simulink model "Loop_detailed_model_comp_cc_vccc_v14_JAWOLL_2"  (R2013a)
settings: Solver=ode15s  SolverMode=SingleTasking  StartTime=0.0  StopTime=8e-3  FixedStep=FS  MaxStep=1e-4  RelTol=1e-3
PreLoadFcn:
  | %lowerVoltageLimit=str2num(get_param(gcs,'lowerVoltageLimit'));
  | %upperVoltageLimit=str2num(get_param(gcs,'upperVoltageLimit'));
InitFcn:
  | %%%%%%  set scope time range
  | T_STOP=str2num(get_param(gcs,'StopTime'));
  | if numel(T_STOP) > 1
  |    T_STOP=T_STOP(2);
  | else
  |    T_STOP=T_STOP(1);
  | end
  | T_STOP=num2str(T_STOP);
  | 
  | %%%%%%  set scope time range in system @init_callback_fct
  | T_STOP=num2str(str2num(get_param(gcs,'StopTime')));
  | 
  | childs = allchild(0);
  | sol=strfind(upper(get(allchild(0),'Tag')),'VIEWER_PARAMETERS');
  | 
  | if iscell(sol)
  |    ind=find(~cellfun(@isempty, strfind(upper(get(allchild(0),'Tag')),'VIEWER_PARAMETERS')));
  | else
  |    ind=sol;
  | end
  | %ind=find(~cellfun(@isempty, {strfind(upper(get(allchild(0),'Tag')),'VIEWER_PARAMETERS'),[]}))
  | if ~isempty(ind)
  |    for k=1:length(childs(ind))
  |       set_param(getfield(get(childs(ind(k)),'UserData'),'block'),'TimeRange', T_STOP);
  | %      get_param(getfield(get(childs(ind(k)),'UserData'),'block'),'TimeRange');
  | %    set_param(getfield(get(childs(ind),'UserData'),'block'),'TimeRange',T_STOP);
  | %    get_param(getfield(get(childs(ind),'UserData'),'block'),'TimeRange');
  |    end
  | else
  |     warning(sprintf('VIEWER_PARAMETERS object not found\nOpen the config dialog by hand for the first sim start'))
  | end
StartFcn:
  | lowerVoltageLimit=str2num(get_param(gcs,'lowerVoltageLimit'));
  | upperVoltageLimit=str2num(get_param(gcs,'upperVoltageLimit'));
model workspace (MATLAB code in the model file):
  | lowerVoltageLimit=str2num(get_param(gcs,'lowerVoltageLimit'));
  | upperVoltageLimit=str2num(get_param(gcs,'upperVoltageLimit'));
values from neighbouring files (symbols this model uses):
  FS = 5e-6    (= 5e-06)    [GalvoModel_v4_sys.m]    (also in GalvoModel_v6_sys.m = 5e-05; Galvo_process_analyze.m = 0.0001)
  Lc = 170e-6    (= 0.00017)    [GalvoModel_v6_sys.m]    (also in Galvo_process_analyze.m)
undefined symbols (not defined in the file or in its folder): ccG0
libraries: simulink x2
settings Model: upperVoltageLimit=30  lowerVoltageLimit=-30  BufferReuse=off  Creator=mainster  LastModifiedBy=mainster
settings SolverCC: AutoInsertRateTranBlk=on
settings OptimizationCC: InlineParams=on  BufferReuse=off
settings DebuggingCC: InitInArrayFormatMsg=none
settings HardwareCC: ProdLargestAtomicInteger=Long  ProdLargestAtomicFloat=Double  ProdEndianess=LittleEndian  ProdHWDeviceType=ARM Compatible->ARM Cortex

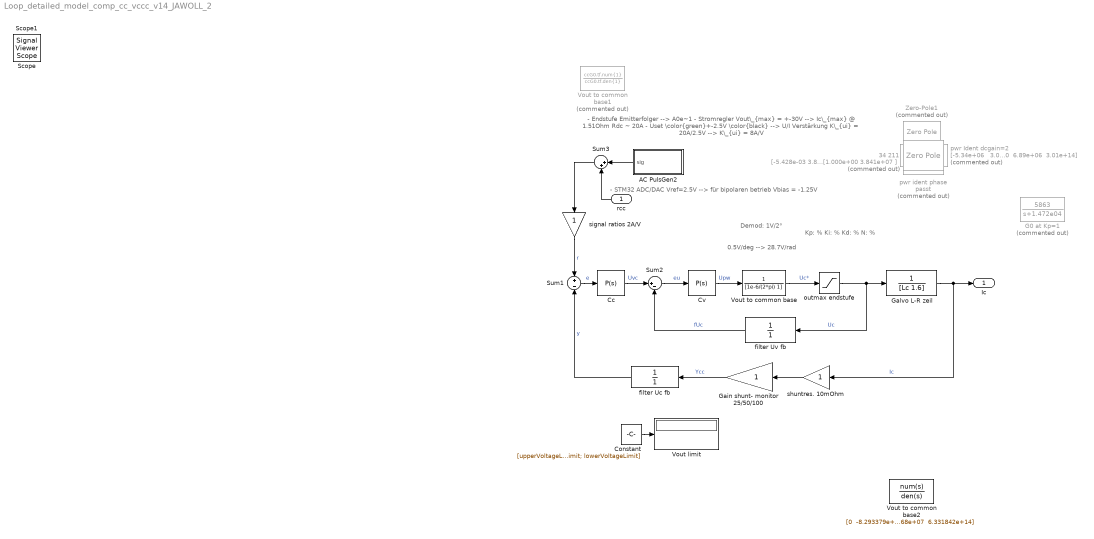
== system Loop_detailed_model_comp_cc_vccc_v14_JAWOLL_2 ==
  note: - Endstufe Emitterfolger --> A0e~1
      | - Stromregler Vout\_{max} = +-30V
      |       --> Ic\_{max} @ 1.51Ohm Rdc ~ 20A
      | - Uset \color{green}+-2.5V \color{black}
      |       --> U/I Verstärkung K\_{ui} = 20A/2.5V
      |       --> K\_{ui} = 8A/V
  note: - STM32 ADC/DAC Vref=2.5V
      | --> für bipolaren betrieb Vbias = -1.25V
  note: Kp: % Ki: % Kd: % N: %
  note: 0.5V/deg --> 28.7V/rad
  note: Demod:
      | 1V/2°
  rcc : Inport
  34 211 : TransferFcn  Commented=on  Numerator=[-5.428e-03 3.828e+07 ]/[-5.428e-03 3.828e+07 ]  Denominator=[1.000e+00 3.841e+07 ]/[1.000e+00 3.841e+07 ]
  AC PulsGen2 : Subsystem  mask{sigp=1, sigpp=0, offs=0}
      mask prompts: sigp "Insert signal peak"; sigpp "or signal peak-to-peak"; offs "Insert DC offset"
      mask TypeOptions sigp: PulsGen/Amplitude
      mask Callback sigp:
      | %sigp=get_param([gcb '/PulsGen'],'Amplitude')
      | %SigVal=2*sigp
      mask TypeOptions offs: offset/Value
      mask Display:
      | %str=sprintf('%s',get(gcbh,'ModelName'));
      | port_label('output', 1, '','texmode','off')
      | %text(.05,.98,['{\fontsize{12}\it\bf' strrep(str,'_',' ') '}'],'horizontalAlignment','left','verticalAlignment','top','texmode','on')
      | %text(.5,0.95,['{\fontsize{8}A_{peak}=}'],'horizontalAlignment','center','verticalAlignment','top','texmode','on')
      | disp(sprintf('Up=%.3g\nDC=%.3g',sigp, offs))
      | %disp(['Upp=' sigpp])%, offs))
      | %sprintf('sigpp==%s',sigpp)
      | %text(.15,.05,['{\fontsize{10}\itmechanics}'],'horizontalAlignment','left','verticalAlignment','bottom','texmode','on')
  Cc : simulink/Continuous/PID Controller  Controller=P  TimeDomain=Continuous-time  SampleTime=1  IntegratorMethod=Forward Euler  FilterMethod=Forward Euler  Form=Parallel  P=10  I=1  D=0  N=100  InitialConditionSource=internal  InitialConditionForIntegrator=0  InitialConditionForFilter=0  ExternalReset=none  LimitOutput=on  UpperSaturationLimit=30  LowerSaturationLimit=-30  LinearizeAsGain=on  AntiWindupMode=none  Kb=1  TrackingMode=off  Kt=1  PParamMin=[]  PParamMax=[]  IParamMin=[]  IParamMax=[]  DParamMin=[]  DParamMax=[]  NParamMin=[]  NParamMax=[]  KbParamMin=[]  KbParamMax=[]  KtParamMin=[]  KtParamMax=[]  POutMin=[]  POutMax=[]  IOutMin=[]  IOutMax=[]  DOutMin=[]  DOutMax=[]  NOutMin=[]  NOutMax=[]  KbOutMin=[]  KbOutMax=[]  KtOutMin=[]  KtOutMax=[]  IntegratorOutMin=[]  IntegratorOutMax=[]  FilterOutMin=[]  FilterOutMax=[]  SumOutMin=[]  SumOutMax=[]  SumI1OutMin=[]  SumI1OutMax=[]  SumI2OutMin=[]  SumI2OutMax=[]  SumI3OutMin=[]  SumI3OutMax=[]  SumDOutMin=[]  SumDOutMax=[]  SaturationOutMin=[]  SaturationOutMax=[]  IntegratorContinuousStateAttributes=''  IntegratorStateMustResolveToSignalObject=off  IntegratorRTWStateStorageClass=Auto  FilterContinuousStateAttributes=''  FilterStateMustResolveToSignalObject=off  FilterRTWStateStorageClass=Auto
      settings: AttributesFormatString=Kpc=%<P>
  Constant : Constant  Value=[upperVoltageLimit; lowerVoltageLimit]
  Cv : simulink/Continuous/PID Controller  Controller=P  TimeDomain=Continuous-time  SampleTime=1  IntegratorMethod=Forward Euler  FilterMethod=Forward Euler  Form=Parallel  P=1  I=1  D=0  N=100  InitialConditionSource=internal  InitialConditionForIntegrator=0  InitialConditionForFilter=0  ExternalReset=none  LimitOutput=on  UpperSaturationLimit=upperVoltageLimit  LowerSaturationLimit=lowerVoltageLimit  LinearizeAsGain=on  AntiWindupMode=none  Kb=1  TrackingMode=off  Kt=1  PParamMin=[]  PParamMax=[]  IParamMin=[]  IParamMax=[]  DParamMin=[]  DParamMax=[]  NParamMin=[]  NParamMax=[]  KbParamMin=[]  KbParamMax=[]  KtParamMin=[]  KtParamMax=[]  POutMin=[]  POutMax=[]  IOutMin=[]  IOutMax=[]  DOutMin=[]  DOutMax=[]  NOutMin=[]  NOutMax=[]  KbOutMin=[]  KbOutMax=[]  KtOutMin=[]  KtOutMax=[]  IntegratorOutMin=[]  IntegratorOutMax=[]  FilterOutMin=[]  FilterOutMax=[]  SumOutMin=[]  SumOutMax=[]  SumI1OutMin=[]  SumI1OutMax=[]  SumI2OutMin=[]  SumI2OutMax=[]  SumI3OutMin=[]  SumI3OutMax=[]  SumDOutMin=[]  SumDOutMax=[]  SaturationOutMin=[]  SaturationOutMax=[]  IntegratorContinuousStateAttributes=''  IntegratorStateMustResolveToSignalObject=off  IntegratorRTWStateStorageClass=Auto  FilterContinuousStateAttributes=''  FilterStateMustResolveToSignalObject=off  FilterRTWStateStorageClass=Auto
      settings: AttributesFormatString=Kpv=%<P>
  G0 at Kp=1 : TransferFcn  Commented=on  Numerator=5863  Denominator="[1  1.472e04]"
  Gain shunt- monitor 25/50/100 : Gain  SampleTime=0
  Galvo L-R zeil : TransferFcn  Numerator=1  Denominator=[Lc 1.6]
  Sum1 : Sum  Inputs=+|-  SampleTime=0
  Sum2 : Sum  Inputs=|+-
  Sum3 : Sum  Inputs=|++  SampleTime=0
  Vout limit : Display
  Vout to common base : TransferFcn  Numerator=1  Denominator=[1e-6/(2*pi) 1]
  Vout to common base1 : TransferFcn  Commented=on  Numerator=ccG0.tf.num{1}  Denominator=ccG0.tf.den{1}
  Vout to common base2 : TransferFcn  Numerator="[0  -8.293379e+06  3.165850e+14]"  Denominator="[1  4.170468e+07  6.331842e+14]"
  Zero-Pole1 : ZeroPole  Commented=on  Zeros=-5.618e7  Poles=[-0.3445+1.7004i -0.3445-1.7004i]
  filter Uc fb : TransferFcn  Denominator=1
  filter Uv fb : TransferFcn  Denominator=1
  outmax endstufe : Saturate  UpperLimit=1000  LowerLimit=-1000
  pwr Ident dcgain=2 : TransferFcn  Commented=on  Numerator="[-5.34e+06   3.00e+14]"  Denominator="[1.00e+00  6.89e+06  3.01e+14]"
  pwr ident phase passt : ZeroPole  Commented=on  Zeros=[]  Poles=[-7.2010 -0.0385]*1e9  Gain=2.76e17
  shuntres. 10mOhm : Gain  SampleTime=0
  signal ratios 2A/V : Gain  SampleTime=0
  Ic : Outport  SampleTime=0
  Scope : SignalViewerScope  IOType=viewer  NumInputPorts=4  ZoomMode=xonly  LegendLocations=|  RefreshTime=0.035000
      | 0.838     0.91933     0.10921    0.021692
      | 0.81634     0.68289     0.13087    0.038639
      | 0.81634     0.46339     0.13087    0.021692
      | 0.81634     0.21109     0.13087    0.038639
      settings: ShowLegends=on  TimeRange=0.015  YMin=-1~-20~-20~-1.5  YMax=1~20~20~1.5
  Scope1 : SignalViewerScope  IOType=viewer  NumInputPorts=4  LegendLocations=|  RefreshTime=0.035000
      | 0.798     0.93887      0.1403    0.020812
      | 0.798     0.70161      0.1403    0.020812
      |     0           0           0           0
      |     0           0           0           0
      settings: ShowLegends=on  TimeRange=0.008  YMin=-40~-8~-5~-5  YMax=40~8~5~5
  wires:
  Galvo L-R zeil/1 -> shuntres. 10mOhm/1, Ic/1  "Ic"
  Cv/1 -> Vout to common base/1  "Upw"
  Vout to common base/1 -> outmax endstufe/1  "Uc*"
  Sum1/1 -> Cc/1  "e"
  Gain shunt- monitor 25/50/100/1 -> filter Uc fb/1  "Ycc"
  shuntres. 10mOhm/1 -> Gain shunt- monitor 25/50/100/1
  signal ratios 2A/V/1 -> Sum1/1  "r"
  Sum2/1 -> Cv/1  "eu"
  Cc/1 -> Sum2/1  "Uvc"
  filter Uv fb/1 -> Sum2/2  "fUc"
  AC PulsGen2/1(sig) -> Sum3/1
  Sum3/1 -> signal ratios 2A/V/1
  rcc/1 -> Sum3/2
  filter Uc fb/1 -> Sum1/2  "y"
  outmax endstufe/1 -> Galvo L-R zeil/1, filter Uv fb/1  "Uc"
  Constant/1 -> Vout limit/1

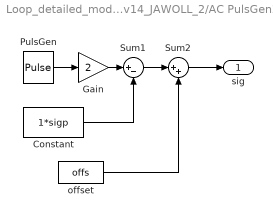
== system Loop_detailed_model_comp_cc_vccc_v14_JAWOLL_2/AC PulsGen2 ==
  Constant : Constant  Value=1*sigp
  Gain : Gain  Gain=2
  PulsGen : DiscretePulseGenerator  PulseType=Time based  Amplitude=sigp  Period=4e-3  PulseWidth=50  PhaseDelay=0.5e-3  SampleTime=FS
      settings: AttributesFormatString=A=%<Amplitude>\nPeri=%<Period>
  Sum1 : Sum  Inputs=|+-
  Sum2 : Sum  Inputs=|++
  offset : Constant  Value=offs
  sig : Outport
  wires:
  Sum2/1 -> sig/1
  PulsGen/1 -> Gain/1
  offset/1 -> Sum2/2
  Gain/1 -> Sum1/1
  Sum1/1 -> Sum2/1
  Constant/1 -> Sum1/2
